simulink model "dtmf_audio_toolbox"  (R2024a)
settings: Solver=FixedStepDiscrete  StartTime=0.0  StopTime=5.5  RelTol=1e-3
PreLoadFcn:
  | load dspafxr;
libraries: dspstat3 x9, dspsrcs4 x8
settings Model: Creator=sv7  LastModifiedBy=johannesarizie
settings SolverCC: AlgebraicLoopSolver=TrustRegion  PositivePriorityOrder=on
settings DataIOCC: SaveFormat=Array  SignalLoggingSaveFormat=ModelDataLogs  SaveOutput=off  SaveTime=off  ReturnWorkspaceOutputs=off
settings OptimizationCC: DefaultParameterBehavior=Inlined  InlineInvariantSignals=on  ExpressionDepthLimit=2147483647  InitFltsAndDblsToZero=on  LifeSpan=1
settings DebuggingCC: SaveWithParameterizedLinksMsg=none  UnderspecifiedInitializationDetection=Classic  MergeDetectMultiDrivingBlocksExec=none  SignalResolutionControl=TryResolveAllWithWarning  SolverPrmCheckMsg=warning  MultiTaskDSMMsg=warning  MultiTaskCondExecSysMsg=none  FcnCallInpInsideContextMsg=warning  UnconnectedInputMsg=warning  UnconnectedOutputMsg=warning  UnconnectedLineMsg=warning  StateNameClashWarn=warning  SFUnexpectedBacktrackingDiag=warning  SFNoUnconditionalDefaultTransitionDiag=warning  ArithmeticOperatorsInVariantConditions=warning
settings HardwareCC: ProdBitPerLong=40  ProdBitPerPointer=32  ProdBitPerSizeT=32  ProdBitPerPtrDiffT=32  ProdLargestAtomicInteger=Integer  ProdLargestAtomicFloat=None  ProdWordSize=32  ProdHWDeviceType=Texas Instruments->C6000  TargetBitPerLong=40  TargetLargestAtomicInteger=Integer  TargetIntDivRoundTo=Zero  TargetEndianess=LittleEndian  TargetHWDeviceType=TI C6000
settings ModelReferenceCC: EnableRefExpFcnMdlSchedulingChecks=on  PropagateSignalLabelsOutOfModel=off
settings SFSimCC: SimUseLocalCustomCode=off  CustomCodeUndefinedFunction=UseInterfaceOnly
settings RTWCC: Description=IDE Link ERT  SystemTargetFile=idelink_ert.tlc  GenerateMakefile=off  TemplateMakefile=none  RTWUseLocalCustomCode=off  GPUComputeCapability=3.5
settings CodeAppCC: StateflowObjectComments=on
settings TargetCC: CompOptLevelCompliant=off  ConcurrentExecutionCompliant=on  CombineOutputUpdateFcns=on  MATLABClassNameForMDSCustomization=linkfoundation.pjtgenerator.IdelinkCustomization  GRTInterface=off  InstructionSetFMA=off  OptimizeReductions=off  LogToMDFFile=off
settings ConfigComp: CovMetricSettings=dw  CovSaveCumulativeToWorkspaceVar=on  CovSaveSingleToWorkspaceVar=on  CovExternalEMLEnable=off
settings TargetHardwareResources: Description=Target Hardware Resources Component

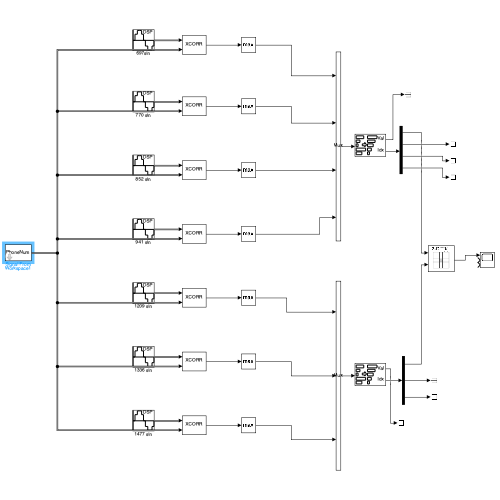
[thumbnail: Simulink's stored preview of the top-level diagram]
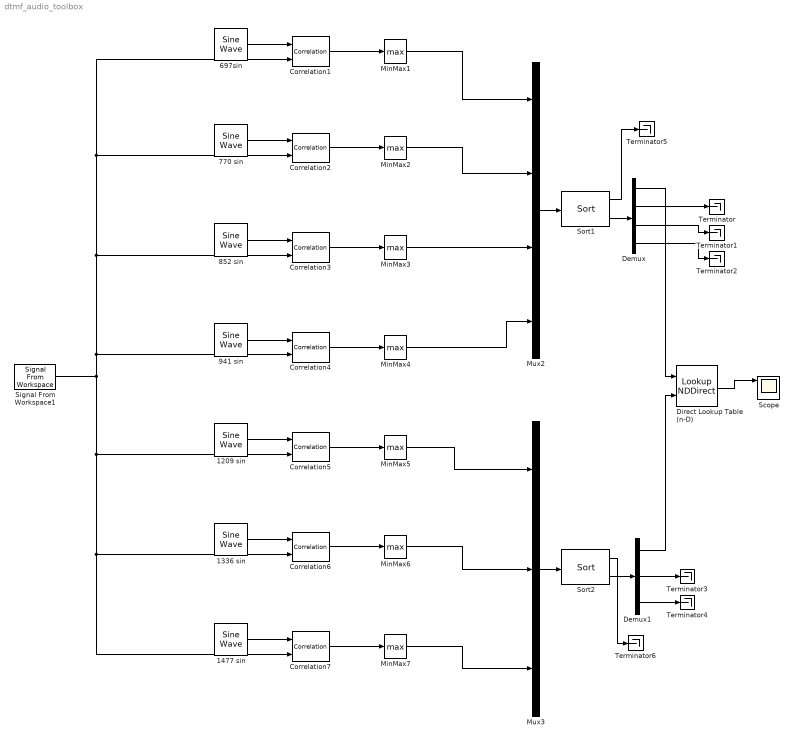
== system dtmf_audio_toolbox ==
  1209 sin : dspsrcs4/Sine Wave  Amplitude=1  Frequency=1209  Phase=0  SampleMode=Discrete  OutComplex=Real  CompMethod=Trigonometric fcn  TableSize=Speed  SampleTime=1/8000  SamplesPerFrame=40  ResetState=Restart at time zero  OutputFrames=on  dataType=double  wordLen=16  udDataType=sfix(16)  fracBitsMode=Best precision  numFracBits=15  OutDataTypeStr=double  LastOutDataTypeStr=double
  1336 sin : dspsrcs4/Sine Wave  Amplitude=1  Frequency=1336  Phase=0  SampleMode=Discrete  OutComplex=Real  CompMethod=Trigonometric fcn  TableSize=Speed  SampleTime=1/8000  SamplesPerFrame=40  ResetState=Restart at time zero  OutputFrames=on  dataType=double  wordLen=16  udDataType=sfix(16)  fracBitsMode=Best precision  numFracBits=15  OutDataTypeStr=double  LastOutDataTypeStr=double
  1477 sin : dspsrcs4/Sine Wave  Amplitude=1  Frequency=1477  Phase=0  SampleMode=Discrete  OutComplex=Real  CompMethod=Trigonometric fcn  TableSize=Speed  SampleTime=1/8000  SamplesPerFrame=40  ResetState=Restart at time zero  OutputFrames=on  dataType=double  wordLen=16  udDataType=sfix(16)  fracBitsMode=Best precision  numFracBits=15  OutDataTypeStr=double  LastOutDataTypeStr=double
  697sin : dspsrcs4/Sine Wave  Amplitude=1  Frequency=697  Phase=0  SampleMode=Discrete  OutComplex=Real  CompMethod=Trigonometric fcn  TableSize=Speed  SampleTime=1/8000  SamplesPerFrame=40  ResetState=Restart at time zero  OutputFrames=on  dataType=double  wordLen=16  udDataType=sfix(16)  fracBitsMode=Best precision  numFracBits=15  OutDataTypeStr=double  LastOutDataTypeStr=double
  770 sin : dspsrcs4/Sine Wave  Amplitude=1  Frequency=770  Phase=0  SampleMode=Discrete  OutComplex=Real  CompMethod=Trigonometric fcn  TableSize=Speed  SampleTime=1/8000  SamplesPerFrame=40  ResetState=Restart at time zero  OutputFrames=on  dataType=double  wordLen=16  udDataType=sfix(16)  fracBitsMode=Best precision  numFracBits=15  OutDataTypeStr=double  LastOutDataTypeStr=double
  852 sin : dspsrcs4/Sine Wave  Amplitude=1  Frequency=852  Phase=0  SampleMode=Discrete  OutComplex=Real  CompMethod=Trigonometric fcn  TableSize=Speed  SampleTime=1/8000  SamplesPerFrame=40  ResetState=Restart at time zero  OutputFrames=on  dataType=double  wordLen=16  udDataType=sfix(16)  fracBitsMode=Best precision  numFracBits=15  OutDataTypeStr=double  LastOutDataTypeStr=double
  941 sin : dspsrcs4/Sine Wave  Amplitude=1  Frequency=941  Phase=0  SampleMode=Discrete  OutComplex=Real  CompMethod=Trigonometric fcn  TableSize=Speed  SampleTime=1/8000  SamplesPerFrame=40  ResetState=Restart at time zero  OutputFrames=on  dataType=double  wordLen=16  udDataType=sfix(16)  fracBitsMode=Best precision  numFracBits=15  OutDataTypeStr=double  LastOutDataTypeStr=double
  Correlation{1..7} (7 alike) : dspstat3/Correlation  domain=Time  roundingMode=Floor  overflowMode=off  outputDataTypeStr=Inherit: Same as accumulator  outputMin=[]  outputMax=[]  outputLastDataTypeStr=Inherit: Same as accumulator
  Demux : Demux
  Demux1 : Demux  Outputs=3
  Direct Lookup Table (n-D) : LookupNDDirect  Table=[0 0 0 0;0 1 2 3; 0 4 5 6; 0 7 8 9; 0 0 0 0]
  MinMax{1..7} (7 alike) : MinMax  Function=max
  Mux2 : Mux
  Mux3 : Mux  Inputs=3
  Scope : Scope  NumInputPorts=3
  Signal From Workspace1 : dspsrcs4/Signal From Workspace  X=PhoneNum  Ts=1/8000  nsamps=40  OutputAfterFinalValue=Cyclic repetition  ignoreOrWarnInputAndFrameLengths=off  OutputFrames=on
  Sort1 : dspstat3/Sort  otype=Value and Index  dir=Descending  sortAlg=Quick sort  roundingMode=Floor  overflowMode=off  accumDataTypeStr=Inherit: Same as product output  accumLastDataTypeStr=Inherit: Same as product output
  Sort2 : dspstat3/Sort  otype=Value and Index  dir=Descending  sortAlg=Quick sort  roundingMode=Floor  overflowMode=off  accumDataTypeStr=Inherit: Same as product output  accumLastDataTypeStr=Inherit: Same as product output
  Terminator{,1..6} (7 alike) : Terminator
  wires:
  MinMax2/1 -> Mux2/2
  MinMax3/1 -> Mux2/3
  941 sin/1 -> Correlation4/1
  Correlation4/1 -> MinMax4/1
  Correlation5/1 -> MinMax5/1
  Correlation2/1 -> MinMax2/1
  MinMax4/1 -> Mux2/4
  1336 sin/1 -> Correlation6/1
  852 sin/1 -> Correlation3/1
  MinMax1/1 -> Mux2/1
  Correlation1/1 -> MinMax1/1
  Correlation3/1 -> MinMax3/1
  770 sin/1 -> Correlation2/1
  697sin/1 -> Correlation1/1
  Mux2/1 -> Sort1/1
  MinMax5/1 -> Mux3/1
  1209 sin/1 -> Correlation5/1
  Correlation6/1 -> MinMax6/1
  MinMax6/1 -> Mux3/2
  Mux3/1 -> Sort2/1
  MinMax7/1 -> Mux3/3
  Correlation7/1 -> MinMax7/1
  1477 sin/1 -> Correlation7/1
  Sort1/2 -> Demux/1
  Demux/1 -> Direct Lookup Table (n-D)/1
  Demux1/1 -> Direct Lookup Table (n-D)/2
  Sort2/2 -> Demux1/1
  Signal From Workspace1/1 -> Correlation4/2, Correlation3/2, Correlation1/2, Correlation2/2, Correlation5/2, Correlation6/2, Correlation7/2
  Demux/2 -> Terminator/1
  Demux/3 -> Terminator1/1
  Demux/4 -> Terminator2/1
  Demux1/3 -> Terminator4/1
  Demux1/2 -> Terminator3/1
  Sort1/1 -> Terminator5/1
  Sort2/1 -> Terminator6/1
  Direct Lookup Table (n-D)/1 -> Scope/1
